simulink model "tensegrity_joint_revolute"  (R2022b)
settings: Solver=VariableStepAuto  StartTime=0.0  StopTime=10.0  RelTol=1e-3
InitFcn:
  | parameters_tensegrity_joint;
  | l0_all=cables_l0(fix, fiz, w, h, b);
  | predpeti=0.95;
values from neighbouring files (symbols this model uses):
  fiz = 0    [tensegrity_joint_revolute_stiffness.m]
undefined symbols (not defined in the file or in its folder): a, b, b_all, h, k_all, w
libraries: sm_lib x30, nesl_utility x25
(part 2 of 2)

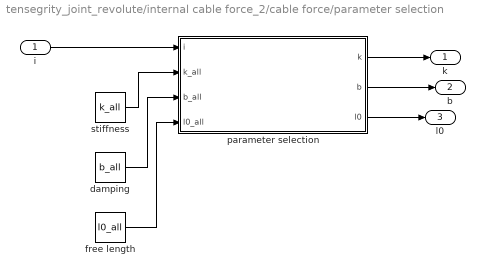
== system tensegrity_joint_revolute/internal cable force_2/cable force/parameter selection ==
  i : Inport
  damping : Constant  Value=b_all
  free length : Constant  Value=l0_all
  parameter selection : MATLAB Function  TreatAsAtomicUnit=on
  stiffness : Constant  Value=k_all
  k : Outport
  b : Outport  Port=2
  l0 : Outport  Port=3
  wires:
  parameter selection/1(k) -> k/1
  parameter selection/3(l0) -> l0/1
  i/1 -> parameter selection/1(i)
  parameter selection/2(b) -> b/1
  free length/1 -> parameter selection/4(l0_all)
  stiffness/1 -> parameter selection/2(k_all)
  damping/1 -> parameter selection/3(b_all)

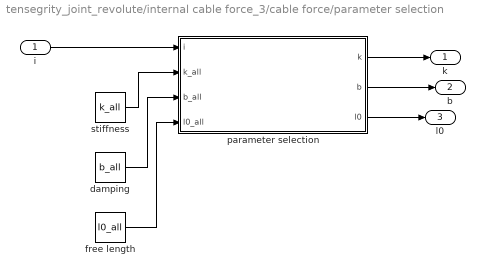
== system tensegrity_joint_revolute/internal cable force_3/cable force/parameter selection ==
  i : Inport
  damping : Constant  Value=b_all
  free length : Constant  Value=l0_all
  parameter selection : MATLAB Function  TreatAsAtomicUnit=on
  stiffness : Constant  Value=k_all
  k : Outport
  b : Outport  Port=2
  l0 : Outport  Port=3
  wires:
  damping/1 -> parameter selection/3(b_all)
  stiffness/1 -> parameter selection/2(k_all)
  free length/1 -> parameter selection/4(l0_all)
  parameter selection/2(b) -> b/1
  i/1 -> parameter selection/1(i)
  parameter selection/3(l0) -> l0/1
  parameter selection/1(k) -> k/1

== system tensegrity_joint_revolute/internal cable force_4/cable force/parameter selection ==
  i : Inport
  damping : Constant  Value=b_all
  free length : Constant  Value=l0_all
  parameter selection : MATLAB Function  TreatAsAtomicUnit=on
  stiffness : Constant  Value=k_all
  k : Outport
  b : Outport  Port=2
  l0 : Outport  Port=3
  wires:
  parameter selection/1(k) -> k/1
  parameter selection/3(l0) -> l0/1
  i/1 -> parameter selection/1(i)
  parameter selection/2(b) -> b/1
  free length/1 -> parameter selection/4(l0_all)
  stiffness/1 -> parameter selection/2(k_all)
  damping/1 -> parameter selection/3(b_all)

== system tensegrity_joint_revolute/internal cable force_5/cable force/parameter selection ==
  i : Inport
  damping : Constant  Value=b_all
  free length : Constant  Value=l0_all
  parameter selection : MATLAB Function  TreatAsAtomicUnit=on
  stiffness : Constant  Value=k_all
  k : Outport
  b : Outport  Port=2
  l0 : Outport  Port=3
  wires:
  parameter selection/1(k) -> k/1
  parameter selection/3(l0) -> l0/1
  i/1 -> parameter selection/1(i)
  parameter selection/2(b) -> b/1
  free length/1 -> parameter selection/4(l0_all)
  stiffness/1 -> parameter selection/2(k_all)
  damping/1 -> parameter selection/3(b_all)

== system tensegrity_joint_revolute/internal cable force_6/cable force/parameter selection ==
  i : Inport
  damping : Constant  Value=b_all
  free length : Constant  Value=l0_all
  parameter selection : MATLAB Function  TreatAsAtomicUnit=on
  stiffness : Constant  Value=k_all
  k : Outport
  b : Outport  Port=2
  l0 : Outport  Port=3
  wires:
  damping/1 -> parameter selection/3(b_all)
  stiffness/1 -> parameter selection/2(k_all)
  free length/1 -> parameter selection/4(l0_all)
  parameter selection/2(b) -> b/1
  i/1 -> parameter selection/1(i)
  parameter selection/3(l0) -> l0/1
  parameter selection/1(k) -> k/1

== system tensegrity_joint_revolute/internal cable force_7/cable force/parameter selection ==
  i : Inport
  damping : Constant  Value=b_all
  free length : Constant  Value=l0_all
  parameter selection : MATLAB Function  TreatAsAtomicUnit=on
  stiffness : Constant  Value=k_all
  k : Outport
  b : Outport  Port=2
  l0 : Outport  Port=3
  wires:
  parameter selection/1(k) -> k/1
  parameter selection/3(l0) -> l0/1
  i/1 -> parameter selection/1(i)
  parameter selection/2(b) -> b/1
  free length/1 -> parameter selection/4(l0_all)
  stiffness/1 -> parameter selection/2(k_all)
  damping/1 -> parameter selection/3(b_all)

== system tensegrity_joint_revolute/internal cable force_8/cable force/parameter selection ==
  i : Inport
  damping : Constant  Value=b_all
  free length : Constant  Value=l0_all
  parameter selection : MATLAB Function  TreatAsAtomicUnit=on
  stiffness : Constant  Value=k_all
  k : Outport
  b : Outport  Port=2
  l0 : Outport  Port=3
  wires:
  damping/1 -> parameter selection/3(b_all)
  stiffness/1 -> parameter selection/2(k_all)
  free length/1 -> parameter selection/4(l0_all)
  parameter selection/2(b) -> b/1
  i/1 -> parameter selection/1(i)
  parameter selection/3(l0) -> l0/1
  parameter selection/1(k) -> k/1

== matlab function tensegrity_joint_revolute/internal cable force_6/cable force/cable force computation ==
  data: k input; Fc output; b input; l0 input; l input; v input
function Fc = cable_force(k, b,l0, l, v)

Fc=k*(l-l0) + b*v;

== matlab function tensegrity_joint_revolute/internal cable force_6/cable force/parameter selection/parameter selection ==
  data: i input; k output; k_all input; b_all input; l0_all input; b output; l0 output
function [k, b, l0] = parameter_selection(i, k_all, b_all, l0_all)

k=k_all(i);
b=b_all(i);
l0=l0_all(i);

== matlab function tensegrity_joint_revolute/internal cable force_2/cable force/cable force computation ==
  data: k input; Fc output; b input; l0 input; l input; v input
function Fc = cable_force(k, b,l0, l, v)

Fc=k*(l-l0) + b*v;

== matlab function tensegrity_joint_revolute/internal cable force_7/cable force/cable force computation ==
  data: k input; Fc output; b input; l0 input; l input; v input
function Fc = cable_force(k, b,l0, l, v)

Fc=k*(l-l0) + b*v;

== matlab function tensegrity_joint_revolute/internal cable force_7/cable force/parameter selection/parameter selection ==
  data: i input; k output; k_all input; b_all input; l0_all input; b output; l0 output
function [k, b, l0] = parameter_selection(i, k_all, b_all, l0_all)

k=k_all(i);
b=b_all(i);
l0=l0_all(i);

== matlab function tensegrity_joint_revolute/internal cable force_8/cable force/cable force computation ==
  data: k input; Fc output; b input; l0 input; l input; v input
function Fc = cable_force(k, b,l0, l, v)

Fc=k*(l-l0) + b*v;

== matlab function tensegrity_joint_revolute/internal cable force_8/cable force/parameter selection/parameter selection ==
  data: i input; k output; k_all input; b_all input; l0_all input; b output; l0 output
function [k, b, l0] = parameter_selection(i, k_all, b_all, l0_all)

k=k_all(i);
b=b_all(i);
l0=l0_all(i);

== matlab function tensegrity_joint_revolute/internal cable force_1/cable force/cable force computation ==
  data: k input; Fc output; b input; l0 input; l input; v input
function Fc = cable_force(k, b,l0, l, v)

Fc=k*(l-l0) + b*v;

== matlab function tensegrity_joint_revolute/internal cable force_1/cable force/parameter selection/parameter selection ==
  data: i input; k output; k_all input; b_all input; l0_all input; b output; l0 output
function [k, b, l0] = parameter_selection(i, k_all, b_all, l0_all)

k=k_all(i);
b=b_all(i);
l0=l0_all(i);

== matlab function tensegrity_joint_revolute/internal cable force_2/cable force/parameter selection/parameter selection ==
  data: i input; k output; k_all input; b_all input; l0_all input; b output; l0 output
function [k, b, l0] = parameter_selection(i, k_all, b_all, l0_all)

k=k_all(i);
b=b_all(i);
l0=l0_all(i);

== matlab function tensegrity_joint_revolute/internal cable force_3/cable force/cable force computation ==
  data: k input; Fc output; b input; l0 input; l input; v input
function Fc = cable_force(k, b,l0, l, v)

Fc=k*(l-l0) + b*v;

== matlab function tensegrity_joint_revolute/internal cable force_3/cable force/parameter selection/parameter selection ==
  data: i input; k output; k_all input; b_all input; l0_all input; b output; l0 output
function [k, b, l0] = parameter_selection(i, k_all, b_all, l0_all)

k=k_all(i);
b=b_all(i);
l0=l0_all(i);

== matlab function tensegrity_joint_revolute/internal cable force_4/cable force/cable force computation ==
  data: k input; Fc output; b input; l0 input; l input; v input
function Fc = cable_force(k, b,l0, l, v)

Fc=k*(l-l0) + b*v;

== matlab function tensegrity_joint_revolute/internal cable force_4/cable force/parameter selection/parameter selection ==
  data: i input; k output; k_all input; b_all input; l0_all input; b output; l0 output
function [k, b, l0] = parameter_selection(i, k_all, b_all, l0_all)

k=k_all(i);
b=b_all(i);
l0=l0_all(i);

== matlab function tensegrity_joint_revolute/internal cable force_5/cable force/cable force computation ==
  data: k input; Fc output; b input; l0 input; l input; v input
function Fc = cable_force(k, b,l0, l, v)

Fc=k*(l-l0) + b*v;

== matlab function tensegrity_joint_revolute/internal cable force_5/cable force/parameter selection/parameter selection ==
  data: i input; k output; k_all input; b_all input; l0_all input; b output; l0 output
function [k, b, l0] = parameter_selection(i, k_all, b_all, l0_all)

k=k_all(i);
b=b_all(i);
l0=l0_all(i);
